simulink model "AsteroidImpact_2018a"  (R2018b)
settings: Solver=ode4  StartTime=0.0  StopTime=45  FixedStep=0.0001  RelTol=1e-3
values from neighbouring files (symbols this model uses):
  g = 9.81    [C_calculation.m]
  m = 10000    [C_calculation.m]
undefined symbols (not defined in the file or in its folder): I, K
libraries: peGeneralControl x6
settings Model: Creator=KNMALE002  LastModifiedBy=Kian
settings DataIOCC: SaveOutput=off  SignalLogging=off  DSMLogging=off  TimeSaveName=simulation_time

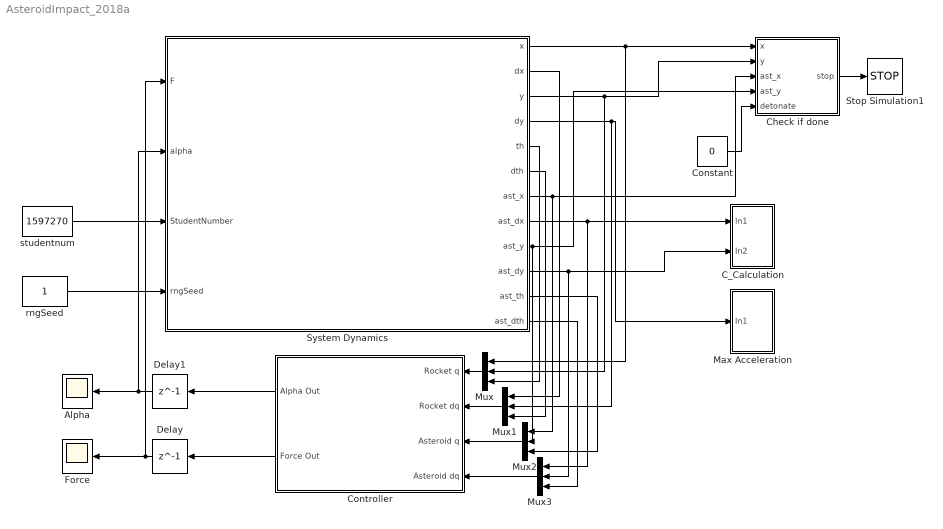
== system AsteroidImpact_2018a ==
  Alpha : Scope
  C_Calculation : Subsystem
  Check if done : MATLAB Function  TreatAsAtomicUnit=on
  Constant : Constant  Value=0
  Controller : Subsystem
  Delay : Delay  DelayLength=1  InitialCondition=10000000000
  Delay1 : Delay  DelayLength=1
  Force : Scope
  Max Acceleration : Subsystem
  Mux{,1..3} (4 alike) : Mux  Inputs=3
  Stop Simulation1 : Stop
  System Dynamics : Subsystem  TreatAsAtomicUnit=on  mask{Value=1}
      mask prompts: Value "Enter mode (1, 2 or 3)"
      mask TypeOptions Value: ScenarioVar/Value
      mask Display: image('lander.jpg');
  rngSeed : Constant
  studentnum : Constant  Value=1597270
  wires:
  studentnum/1 -> System Dynamics/3(StudentNumber)
  System Dynamics/1(x) -> Mux/1, Check if done/1(x)
  rngSeed/1 -> System Dynamics/4(rngSeed)
  System Dynamics/3(y) -> Check if done/2(y), Mux/2
  System Dynamics/7(ast_x) -> Mux2/1, Check if done/3(ast_x)
  System Dynamics/9(ast_y) -> Mux2/2, Check if done/4(ast_y)
  Check if done/1(stop) -> Stop Simulation1/1
  Delay1/1 -> System Dynamics/2(alpha), Alpha/1
  Constant/1 -> Check if done/5(detonate)
  System Dynamics/5(th) -> Mux/3
  System Dynamics/2(dx) -> Mux1/1
  System Dynamics/6(dth) -> Mux1/3
  System Dynamics/8(ast_dx) -> Mux3/1, C_Calculation/1(In1)
  System Dynamics/10(ast_dy) -> Mux3/2, C_Calculation/2(In2)
  System Dynamics/4(dy) -> Max Acceleration/1(In1), Mux1/2
  Mux/1 -> Controller/1(Rocket q)
  Mux1/1 -> Controller/2(Rocket dq)
  Mux2/1 -> Controller/3(Asteroid q)
  Mux3/1 -> Controller/4(Asteroid dq)
  System Dynamics/11(ast_th) -> Mux2/3
  System Dynamics/12(ast_dth) -> Mux3/3
  Delay/1 -> System Dynamics/1(F), Force/1
  Controller/1(Alpha Out) -> Delay1/1
  Controller/2(Force Out) -> Delay/1

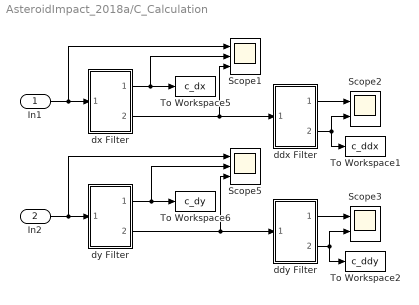
== system AsteroidImpact_2018a/C_Calculation ==
  In1 : Inport
  In2 : Inport  Port=2
  Scope1 : Scope  NumInputPorts=3
  Scope2 : Scope  NumInputPorts=2
  Scope3 : Scope  NumInputPorts=2
  Scope5 : Scope  NumInputPorts=3
  To Workspace1 : ToWorkspace  VariableName=c_ddx  SampleTime=-1
      settings: Save2DSignal=2-D array (concatenate along first dimension)
  To Workspace2 : ToWorkspace  VariableName=c_ddy  SampleTime=-1
      settings: Save2DSignal=2-D array (concatenate along first dimension)
  To Workspace5 : ToWorkspace  VariableName=c_dx  SampleTime=-1
  To Workspace6 : ToWorkspace  VariableName=c_dy  SampleTime=-1
  ddx Filter : Subsystem
  ddy Filter : Subsystem
  dx Filter : Subsystem
  dy Filter : Subsystem
  wires:
  In2/1 -> Scope5/1, dy Filter/1(In1)
  In1/1 -> Scope1/1, dx Filter/1(In1)
  ddy Filter/1(Out1) -> Scope3/1
  ddy Filter/2(Out2) -> To Workspace2/1, Scope3/2
  dy Filter/1(Out1) -> To Workspace6/1, Scope5/2
  dy Filter/2(Out2) -> ddy Filter/1(In1), Scope5/3
  dx Filter/2(Out2) -> ddx Filter/1(In1), Scope1/3
  dx Filter/1(Out1) -> Scope1/2, To Workspace5/1
  ddx Filter/2(Out2) -> To Workspace1/1, Scope2/2
  ddx Filter/1(Out1) -> Scope2/1

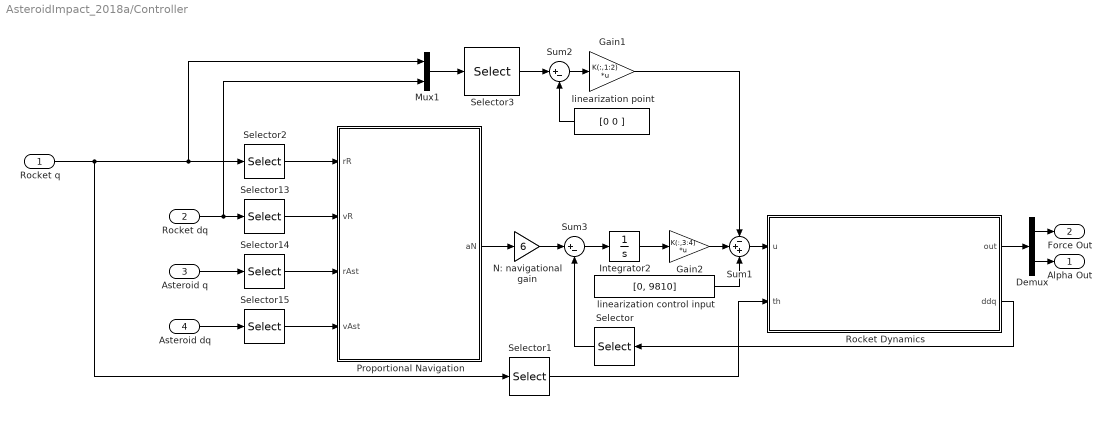
== system AsteroidImpact_2018a/Controller ==
  Rocket q : Inport
  Rocket dq : Inport  Port=2
  Asteroid q : Inport  Port=3
  Asteroid dq : Inport  Port=4
  Demux : Demux  Outputs=2
  Gain1 : Gain  Gain=K(:,1:2)  Multiplication=Matrix(K*u)
  Gain2 : Gain  Gain=K(:,3:4)  Multiplication=Matrix(K*u)
  Integrator2 : Integrator
  Mux1 : Mux  Inputs=2
  N: navigational gain : Gain  Gain=6
  Proportional Navigation : MATLAB Function  TreatAsAtomicUnit=on
  Rocket Dynamics : MATLAB Function  TreatAsAtomicUnit=on
  Selector{,2,13..15} (5 alike) : Selector  InputPortWidth=3  IndexOptions=Index vector (dialog)  Indices=[1 2]  OutputSizes=1
  Selector1 : Selector  InputPortWidth=3  IndexOptions=Index vector (dialog)  Indices=3  OutputSizes=1
  Selector3 : Selector  InputPortWidth=6  IndexOptions=Index vector (dialog)  Indices=[3 6]  OutputSizes=1
  Sum1 : Sum  Inputs=-++
  Sum2 : Sum  Inputs=|+-
  Sum3 : Sum  Inputs=|+-
  linearization control input : Constant  Value=[0, 9810]
  linearization point : Constant  Value=[0 0 ]
  Alpha Out : Outport
  Force Out : Outport  Port=2
  wires:
  Selector15/1 -> Proportional Navigation/4(vAst)
  Rocket dq/1 -> Mux1/2, Selector13/1
  Selector13/1 -> Proportional Navigation/2(vR)
  Selector14/1 -> Proportional Navigation/3(rAst)
  Proportional Navigation/1(aN) -> N: navigational gain/1
  Rocket Dynamics/2(ddq) -> Selector/1
  Demux/1 -> Force Out/1
  Selector2/1 -> Proportional Navigation/1(rR)
  Demux/2 -> Alpha Out/1
  Rocket q/1 -> Selector1/1, Mux1/1, Selector2/1
  Mux1/1 -> Selector3/1
  Sum2/1 -> Gain1/1
  linearization control input/1 -> Sum1/3
  Gain1/1 -> Sum1/1
  Selector/1 -> Sum3/2
  Gain2/1 -> Sum1/2
  Sum3/1 -> Integrator2/1
  Integrator2/1 -> Gain2/1
  Asteroid q/1 -> Selector14/1
  Asteroid dq/1 -> Selector15/1
  N: navigational gain/1 -> Sum3/1
  Sum1/1 -> Rocket Dynamics/1(u)
  Selector1/1 -> Rocket Dynamics/2(th)
  Rocket Dynamics/1(out) -> Demux/1
  Selector3/1 -> Sum2/1
  linearization point/1 -> Sum2/2

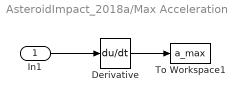
== system AsteroidImpact_2018a/Max Acceleration ==
  In1 : Inport
  Derivative : Derivative
  To Workspace1 : ToWorkspace  VariableName=a_max  SampleTime=-1
      settings: Save2DSignal=2-D array (concatenate along first dimension)
  wires:
  In1/1 -> Derivative/1
  Derivative/1 -> To Workspace1/1

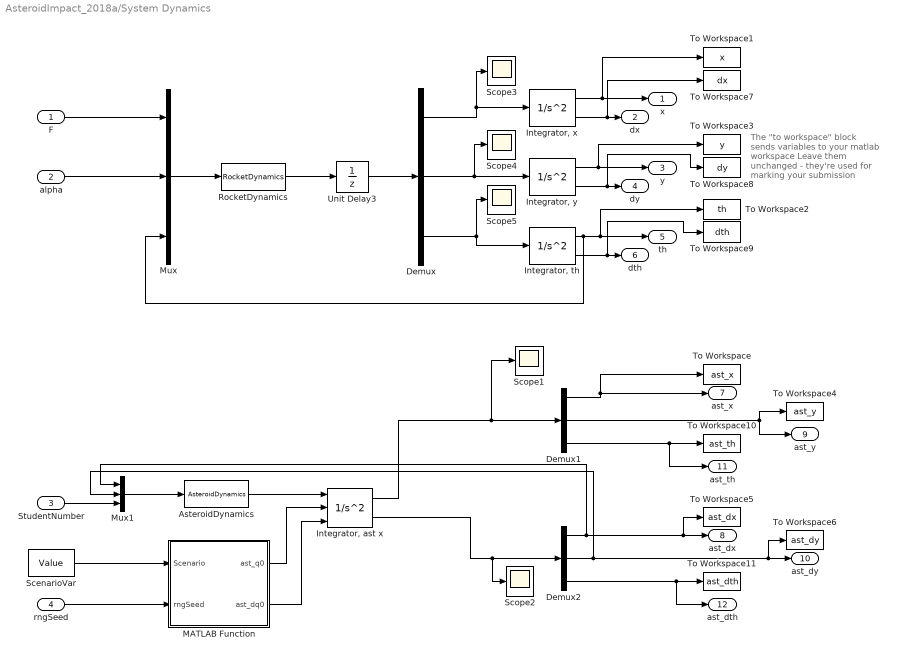
== system AsteroidImpact_2018a/System Dynamics ==
  note: The "to workspace" block sends variables to your matlab workspace
      |
      | Leave them unchanged - they're used for marking your submission
  F : Inport
  alpha : Inport  Port=2
  StudentNumber : Inport  Port=3
  rngSeed : Inport  Port=4
  AsteroidDynamics : MATLABFcn  MATLABFcn=AsteroidDynamics  OutputDimensions=3
  Demux : Demux  Outputs=3
  Demux1 : Demux  Outputs=3
  Demux2 : Demux  Outputs=3
  "Integrator, th" : SecondOrderIntegrator  ICX=0  ICDXDT=0
  "Integrator, x" : SecondOrderIntegrator  ICX=0
  "Integrator, y" : SecondOrderIntegrator  ICX=0
  "Integrator, ast x" : SecondOrderIntegrator  ICSourceX=external  ICX=x0  ICSourceDXDT=external
  MATLAB Function : MATLAB Function  TreatAsAtomicUnit=on
  Mux : Mux  Inputs=3
  Mux1 : Mux  Inputs=3
  RocketDynamics : MATLABFcn  MATLABFcn=RocketDynamics  Output1D=off
  ScenarioVar : Constant  Value=Value
  Scope{1..5} (5 alike) : Scope
  To Workspace : ToWorkspace  VariableName=ast_x  SampleTime=-1
  To Workspace1 : ToWorkspace  VariableName=x  SampleTime=-1
  To Workspace10 : ToWorkspace  VariableName=ast_th  SampleTime=-1
  To Workspace11 : ToWorkspace  VariableName=ast_dth  SampleTime=-1
  To Workspace2 : ToWorkspace  VariableName=th  SampleTime=-1
  To Workspace3 : ToWorkspace  VariableName=y  SampleTime=-1
  To Workspace4 : ToWorkspace  VariableName=ast_y  SampleTime=-1
  To Workspace5 : ToWorkspace  VariableName=ast_dx  SampleTime=-1
  To Workspace6 : ToWorkspace  VariableName=ast_dy  SampleTime=-1
  To Workspace7 : ToWorkspace  VariableName=dx  SampleTime=-1
  To Workspace8 : ToWorkspace  VariableName=dy  SampleTime=-1
  To Workspace9 : ToWorkspace  VariableName=dth  SampleTime=-1
  Unit Delay3 : UnitDelay  SampleTime=-1
  x : Outport  PortDimensions=1
  dx : Outport  Port=2  PortDimensions=1
  y : Outport  Port=3  PortDimensions=1
  dy : Outport  Port=4  PortDimensions=1
  th : Outport  Port=5  PortDimensions=1
  dth : Outport  Port=6  PortDimensions=1
  ast_x : Outport  Port=7  PortDimensions=1
  ast_dx : Outport  Port=8  PortDimensions=1
  ast_y : Outport  Port=9  PortDimensions=1
  ast_dy : Outport  Port=10  PortDimensions=1
  ast_th : Outport  Port=11  PortDimensions=1
  ast_dth : Outport  Port=12  PortDimensions=1
  wires:
  "Integrator, th"/1 -> th/1, To Workspace2/1, Mux/3
  Demux/1 -> Scope3/1, "Integrator, x"/1
  Demux/2 -> Scope4/1, "Integrator, y"/1
  Demux/3 -> "Integrator, th"/1, Scope5/1
  "Integrator, x"/1 -> x/1, To Workspace1/1
  "Integrator, x"/2 -> To Workspace7/1, dx/1
  "Integrator, y"/2 -> To Workspace8/1, dy/1
  "Integrator, th"/2 -> To Workspace9/1, dth/1
  Mux/1 -> RocketDynamics/1
  RocketDynamics/1 -> Unit Delay3/1
  rngSeed/1 -> MATLAB Function/2(rngSeed)
  ScenarioVar/1 -> MATLAB Function/1(Scenario)
  F/1 -> Mux/1
  alpha/1 -> Mux/2
  Demux1/2 -> To Workspace4/1, ast_y/1
  Demux1/3 -> To Workspace10/1, ast_th/1
  Demux2/3 -> ast_dth/1, To Workspace11/1
  Mux1/1 -> AsteroidDynamics/1
  AsteroidDynamics/1 -> "Integrator, ast x"/1
  "Integrator, ast x"/1 -> Scope1/1, Demux1/1
  "Integrator, ast x"/2 -> Scope2/1, Demux2/1
  Demux2/1 -> Mux1/1, To Workspace5/1, ast_dx/1
  Demux2/2 -> Mux1/2, To Workspace6/1, ast_dy/1
  MATLAB Function/1(ast_q0) -> "Integrator, ast x"/2
  MATLAB Function/2(ast_dq0) -> "Integrator, ast x"/3
  StudentNumber/1 -> Mux1/3
  Unit Delay3/1 -> Demux/1
  "Integrator, y"/1 -> y/1, To Workspace3/1
  Demux1/1 -> To Workspace/1, ast_x/1

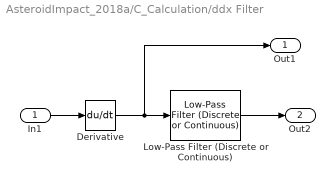
== system AsteroidImpact_2018a/C_Calculation/ddx Filter ==
  In1 : Inport
  Derivative : Derivative
  Low-Pass Filter (Discrete or Continuous) : peGeneralControl/Low-Pass Filter (Discrete or Continuous)  K=1  T=.15  B=inf  A=-inf  Ts=-1
  Out1 : Outport
  Out2 : Outport  Port=2
  wires:
  Low-Pass Filter (Discrete or Continuous)/1 -> Out2/1
  In1/1 -> Derivative/1
  Derivative/1 -> Low-Pass Filter (Discrete or Continuous)/1, Out1/1

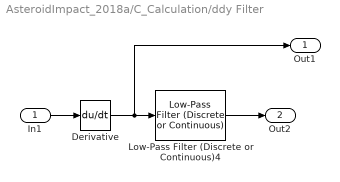
== system AsteroidImpact_2018a/C_Calculation/ddy Filter ==
  In1 : Inport
  Derivative : Derivative
  Low-Pass Filter (Discrete or Continuous)4 : peGeneralControl/Low-Pass Filter (Discrete or Continuous)  K=1  T=.1  B=inf  A=-inf  Ts=-1
  Out1 : Outport
  Out2 : Outport  Port=2
  wires:
  In1/1 -> Derivative/1
  Low-Pass Filter (Discrete or Continuous)4/1 -> Out2/1
  Derivative/1 -> Low-Pass Filter (Discrete or Continuous)4/1, Out1/1

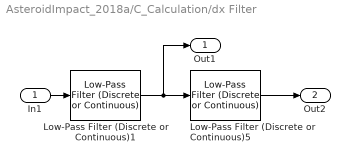
== system AsteroidImpact_2018a/C_Calculation/dx Filter ==
  In1 : Inport
  Low-Pass Filter (Discrete or Continuous)1 : peGeneralControl/Low-Pass Filter (Discrete or Continuous)  K=1  T=0.1  B=inf  A=-inf  Ts=-1
  Low-Pass Filter (Discrete or Continuous)5 : peGeneralControl/Low-Pass Filter (Discrete or Continuous)  K=1  T=0.3  B=inf  A=-inf  Ts=-1
  Out1 : Outport
  Out2 : Outport  Port=2
  wires:
  In1/1 -> Low-Pass Filter (Discrete or Continuous)1/1
  Low-Pass Filter (Discrete or Continuous)1/1 -> Low-Pass Filter (Discrete or Continuous)5/1, Out1/1
  Low-Pass Filter (Discrete or Continuous)5/1 -> Out2/1

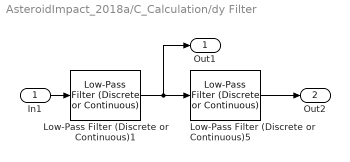
== system AsteroidImpact_2018a/C_Calculation/dy Filter ==
  In1 : Inport
  Low-Pass Filter (Discrete or Continuous)1 : peGeneralControl/Low-Pass Filter (Discrete or Continuous)  K=1  T=.1  B=inf  A=-inf  Ts=-1
  Low-Pass Filter (Discrete or Continuous)5 : peGeneralControl/Low-Pass Filter (Discrete or Continuous)  K=1  T=.3  B=inf  A=-inf  Ts=-1
  Out1 : Outport
  Out2 : Outport  Port=2
  wires:
  In1/1 -> Low-Pass Filter (Discrete or Continuous)1/1
  Low-Pass Filter (Discrete or Continuous)1/1 -> Low-Pass Filter (Discrete or Continuous)5/1, Out1/1
  Low-Pass Filter (Discrete or Continuous)5/1 -> Out2/1

== matlab function AsteroidImpact_2018a/System Dynamics/MATLAB Function ==
  data: ast_q0 output; ast_dq0 output; Scenario input; rngSeed input
function [ast_q0, ast_dq0] = fcn(Scenario, rngSeed)
rng(rngSeed);

if (Scenario == 1)
    x0 = -3000;
    y0 =  5000;
    th0 =   0;
    dx0 = 182;
    dy0 = 0;
    dth0 = 0;

elseif (Scenario == 2)
    x0 = -2000 + rand_within_plus_minus(100);
    y0 = 4000 + rand_within_plus_minus(100); 
    th0 = 0;
    dx0 = 170;
    dy0 = 0;
    dth0 = 0.1;

elseif (Scenario == 3)
    x0 = -2500;
    y0 = 3000;
    th0 = 0;
    dx0 = 160;
    dy0 = 100;
    dth0 = deg2rad(rand_within_plus_minus(20)); % rad/sec

else
    error('You entered an invalid mode -- make sure Scenario = 1, 2 or 3')
end

ast_q0  = [ x0;  y0;  th0];
ast_dq0 = [dx0; dy0; dth0];

end

% calling rand_within_plus_minus(100) returns a number between -100 and 100
function n = rand_within_plus_minus(interval)
    n = (rand - 0.5) * 2 * interval;
end

== matlab function AsteroidImpact_2018a/Controller/Rocket Dynamics ==
  data: out output; u input; ddq output; th input; m parameter; I parameter; g parameter
function [out, ddq]= rDyn(u,th, m, I, g)

F1 = u(1);
F2 = u(2);

ddq = [(F1*cos(th) - F2*sin(th))/m;
 (F2*cos(th) - g*m + F1*sin(th))/m;
 (7*F1)/(2*I)];

F_2 = sqrt(F1^2+F2^2);
ang = atan(-F1/F2);

out = [F_2; ang];

% if mode==1||mode==2
%     out = [30000; atan(-F1/F2)];    
% else
%     F_2 = sqrt(F1^2+F2^2);
%     ang = atan(-F1/F2);
% 
%     out = [F_2; ang];
% end

== matlab function AsteroidImpact_2018a/Check if done ==
  data: x input; stop output; y input; ast_x input; ast_y input; detonate input
function stop = fcn(x, y, ast_x, ast_y, detonate)
    % given the signal to detonate
    if detonate == 1
        stop = 1;

    % rocket has hit the asteroid
    elseif norm([x; y] - [ast_x; ast_y]) < 100
        stop = 1;
    % rocket has hit the ground OR asteroid is close to they city
    elseif y < 0 || ast_y < 200
        stop = 1;
    
    else
        stop = 0;
    end
end

== matlab function AsteroidImpact_2018a/Controller/Proportional Navigation ==
  data: aN output; rR input; vR input; rAst input; vAst input
function aN  = pNav(rR, vR, rAst, vAst)
rT = rAst;
vT = vAst;
rQ = rR;
vQ = vR;

R = rT - rQ;
Rtemp = [R; 0];
V = vT - vQ;
Vtemp = [V; 0];
omega = cross(Rtemp, Vtemp) / dot(Rtemp, Rtemp);
temp = cross(Vtemp, omega);

aN = temp(1:2);
